simulink model "SimScapeMATE_InductionMachine"  (R2024b)
settings: Solver=FixedStepDiscrete  StartTime=0.0  StopTime=0.5  FixedStep=Ts  RelTol=1e-4
PostLoadFcn:
  | Ts=25e-6;
InitFcn:
  | Ts=25e-6;
undefined symbols (not defined in the file): DiscIntNeverNeededParam
libraries: fl_lib x26, ee_lib x16, nesl_utility x13, spspowerguiLib x1
Description:
  | Copyright 2008-2010 The MathWorks, Inc.
settings Model: ARTEMISmethode_block_infos=$$__separator__$$  Creator=MathWorks  LastModifiedBy=CD8435
settings SolverCC: ZeroCrossAlgorithm=Adaptive  AlgebraicLoopSolver=TrustRegion
settings DataIOCC: SaveFormat=Array  SignalLoggingSaveFormat=ModelDataLogs  ReturnWorkspaceOutputs=off  SignalLoggingName=sigsOut  OutputTimes=[0:1/20:10]
settings OptimizationCC: BlockReduction=off  BooleanDataType=off  ExpressionDepthLimit=2147483647  InitFltsAndDblsToZero=on  EfficientMapNaN2IntZero=off  LifeSpan=inf
settings DebuggingCC: UnderspecifiedInitializationDetection=Classic  MergeDetectMultiDrivingBlocksExec=none  CheckExecutionContextPreStartOutputMsg=on  SignalResolutionControl=TryResolveAllWithWarning  IgnoredZcDiagnostic=none  MultiTaskDSMMsg=warning  MultiTaskCondExecSysMsg=none  SigSpecEnsureSampleTimeMsg=none  FcnCallInpInsideContextMsg=warning  AllowSymbolicDim=off  StateNameClashWarn=warning  SFUnexpectedBacktrackingDiag=warning  SFNoUnconditionalDefaultTransitionDiag=warning  SFExecutionAtInitializationDiag=none  ArithmeticOperatorsInVariantConditions=warning
settings HardwareCC: ProdBitPerPointer=32  ProdBitPerSizeT=32  ProdBitPerPtrDiffT=32  ProdLargestAtomicFloat=None  ProdIntDivRoundTo=Undefined  ProdEndianess=Unspecified  ProdWordSize=32  ProdHWDeviceType=Specified  TargetUnknown=on
settings ModelReferenceCC: EnableRefExpFcnMdlSchedulingChecks=on  PropagateSignalLabelsOutOfModel=off
settings SFSimCC: SimUseLocalCustomCode=off  CustomCodeUndefinedFunction=UseInterfaceOnly
settings RTWCC: RTWUseLocalCustomCode=off  GPUComputeCapability=3.5
settings CodeAppCC: StateflowObjectComments=on
settings GRTTargetCC: TargetFcnLib=ansi_tfl_tmw.mat  TargetLangStandard=C89/C90 (ANSI)  CombineOutputUpdateFcns=off  GRTInterface=on
settings ConfigComp: CovMetricSettings=dw  CovSaveCumulativeToWorkspaceVar=on  CovSaveSingleToWorkspaceVar=on  CovExternalEMLEnable=off
settings SimscapeCC: SimscapeNormalizeSystem=off

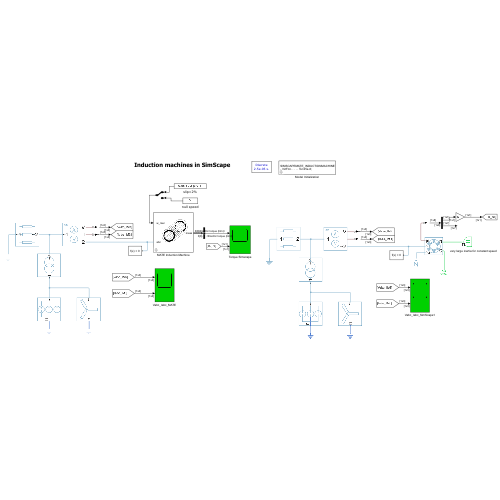
[thumbnail: Simulink's stored preview of the top-level diagram]
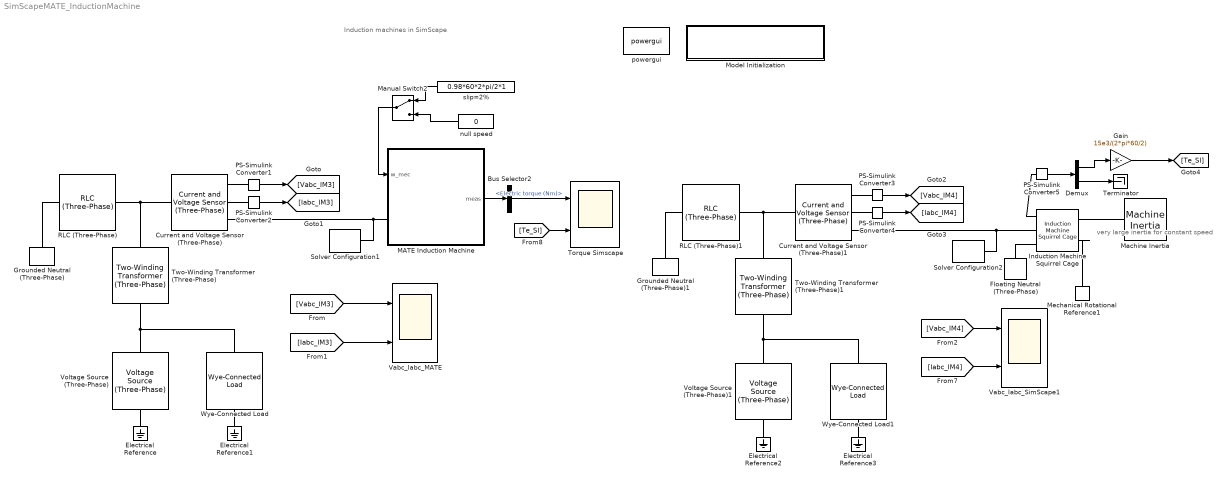
== system SimScapeMATE_InductionMachine ==
  note: very large inertia for constant speed
  note: Induction machines in SimScape
  Bus Selector2 : BusSelector  OutputSignals=Electric torque (Nm)
  Current and Voltage Sensor (Three-Phase) : ee_lib/Sensors & Transducers/Current and Voltage Sensor (Three-Phase)  vMeasurementType=ee.enum.vmeasurement.lg  outputUnit=ee.enum.unit.si  SRated=100e6 A*V  VRated=24e3 V  I_specify=off  I_priority=None  I=[0, 0, 0] A  I_nominal_specify=off  I_nominal_value=1  I_nominal_unit=A  V_specify=off  V_priority=None  V=[0, 0, 0] V  V_nominal_specify=off  V_nominal_value=1  V_nominal_unit=V
      settings: InternalSimscapePortConfiguration="{\"Bottom\":[],\"Left\":[{\"id\":\"N1\",\"label\":\"~1\",\"type\":\"foundation.electrical.three_phase\"}],\"Right\":[{\"id\":\"V_output\",\"label\":\"V\",\"type\":\"output\"},{\"id\":\"I_output\",\"label\":\"I\",\"type\":\"output\"},{\"id\":\"N2\",\"label\":\"~2\",\"type\":\"foundation.electrical.three_phase\"}],\"Top\":[]}"
  Current and Voltage Sensor (Three-Phase)1 : ee_lib/Sensors & Transducers/Current and Voltage Sensor (Three-Phase)  vMeasurementType=ee.enum.vmeasurement.lg  outputUnit=ee.enum.unit.si  SRated=100e6 A*V  VRated=24e3 V  I_specify=off  I_priority=None  I=[0, 0, 0] A  I_nominal_specify=off  I_nominal_value=1  I_nominal_unit=A  V_specify=off  V_priority=None  V=[0, 0, 0] V  V_nominal_specify=off  V_nominal_value=1  V_nominal_unit=V
      settings: InternalSimscapePortConfiguration="{\"Bottom\":[],\"Left\":[{\"id\":\"N1\",\"label\":\"~1\",\"type\":\"foundation.electrical.three_phase\"}],\"Right\":[{\"id\":\"V_output\",\"label\":\"V\",\"type\":\"output\"},{\"id\":\"I_output\",\"label\":\"I\",\"type\":\"output\"},{\"id\":\"N2\",\"label\":\"~2\",\"type\":\"foundation.electrical.three_phase\"}],\"Top\":[]}"
  Demux : Demux  Outputs=[1 -1]
  Electrical Reference{,1..3} (4 alike) : fl_lib/Electrical/Electrical Elements/Electrical Reference
  Floating Neutral (Three-Phase) : ee_lib/Connectors & References/Floating Neutral (Three-Phase)  G_parasitic=1e-12 1/Ohm
      settings: InternalSimscapePortConfiguration="{\"Bottom\":[],\"Left\":[{\"id\":\"N\",\"label\":\"~\",\"type\":\"foundation.electrical.three_phase\"}],\"Right\":[],\"Top\":[]}"
  Gain : Gain  Gain=15e3/(2*pi*60/2)
  Grounded Neutral (Three-Phase) : ee_lib/Connectors & References/Grounded Neutral (Three-Phase)
  Grounded Neutral (Three-Phase)1 : ee_lib/Connectors & References/Grounded Neutral (Three-Phase)
  Induction Machine Squirrel Cage : ee_lib/Electromechanical/Asynchronous/Induction Machine Squirrel Cage  port_option=ee.enum.threePhasePort.composite  SRated=15e3 A*V  VRated=220 V  FRated=60 Hz  nPolePairs=2  param_unit=ee.enum.unit.si  squirrel_cage=ee.enum.squirrelcage.Single  zero_sequence=ee.enum.park.zerosequence.exclude  initialization_option=ee.enum.asm.initialization.fluxvariables  Rs=0.5968 Ohm  Xls=0.0003495*(2*pi*60) Ohm  pu_Rs=0.0258  pu_Lls=0.0413  Rrd=0.6258 Ohm  Xlrd=0.005473*(2*pi*60) Ohm  pu_Rrd=0.0145  pu_Llrd=0.0424  Rrd1=0.28 Ohm  Xlrd1=0.82 Ohm  Rrd2=0.28 Ohm  Xlrd2=0.82 Ohm  pu_Rrd1=0.0290  pu_Llrd1=0.0848  pu_Rrd2=0.0290  pu_Llrd2=0.0848  Xm=0.0354*(2*pi*60) Ohm  pu_Lm=1.7562  X0=0.4 Ohm  pu_L0=0.0413  saturation_option=ee.enum.saturation.exclude  saturation_i=[0, 4, 9, 18, 25, 34, 50, 68, 95, 120] A  saturation_v=[0, 88, 154, 198, 220, 242, 264, 286, 308, 327] V  pu_saturation_i=[0, .176, .396, .792, 1.1, 1.496, 2.2, 2.992, 4.18, 5.28]  pu_saturation_v=[0, .4, .7, .9, 1, 1.1, 1.2, 1.3, 1.4, 1.4864]  connection_option=ee.enum.Connection.delta  angular_position_specify=off  angular_position_priority=None  angular_position=0 deg  angular_position_nominal_specify=off  angular_position_nominal_value=1  angular_position_nominal_unit=deg  pu_psids_specify=off  pu_psids_priority=None  pu_psids=0  pu_psids_nominal_specify=off  pu_psids_nominal_value=1  pu_psids_nominal_unit=1  pu_psiqs_specify=off  pu_psiqs_priority=None  pu_psiqs=0  pu_psiqs_nominal_specify=off  pu_psiqs_nominal_value=1  pu_psiqs_nominal_unit=1  pu_psi0s_specify=off  pu_psi0s_priority=None  pu_psi0s=0  pu_psi0s_nominal_specify=off  pu_psi0s_nominal_value=1  pu_psi0s_nominal_unit=1  pu_psidr_specify=off  pu_psidr_priority=None  pu_psidr=0  pu_psidr_nominal_specify=off  pu_psidr_nominal_value=1  pu_psidr_nominal_unit=1  pu_psiqr_specify=off  pu_psiqr_priority=None  pu_psiqr=0  pu_psiqr_nominal_specify=off  pu_psiqr_nominal_value=1  pu_psiqr_nominal_unit=1  pu_psidr1_specify=off  pu_psidr1_priority=None  pu_psidr1=0  pu_psidr1_nominal_specify=off  pu_psidr1_nominal_value=1  pu_psidr1_nominal_unit=1  pu_psiqr1_specify=off  pu_psiqr1_priority=None  pu_psiqr1=0  pu_psiqr1_nominal_specify=off  pu_psiqr1_nominal_value=1  pu_psiqr1_nominal_unit=1  pu_psidr2_specify=off  pu_psidr2_priority=None  pu_psidr2=0  pu_psidr2_nominal_specify=off  pu_psidr2_nominal_value=1  pu_psidr2_nominal_unit=1  pu_psiqr2_specify=off  pu_psiqr2_priority=None  pu_psiqr2=0  pu_psiqr2_nominal_specify=off  pu_psiqr2_nominal_value=1  pu_psiqr2_nominal_unit=1  psids_specify=off  psids_priority=None  psids=0 Wb  psids_nominal_specify=off  psids_nominal_value=1  psids_nominal_unit=Wb  psiqs_specify=off  psiqs_priority=None  psiqs=0 Wb  psiqs_nominal_specify=off  psiqs_nominal_value=1  psiqs_nominal_unit=Wb  psi0s_specify=off  psi0s_priority=None  psi0s=0 Wb  psi0s_nominal_specify=off  psi0s_nominal_value=1  psi0s_nominal_unit=Wb  psidr_specify=off  psidr_priority=None  psidr=0 Wb  psidr_nominal_specify=off  psidr_nominal_value=1  psidr_nominal_unit=Wb  psiqr_specify=off  psiqr_priority=None  psiqr=0 Wb  psiqr_nominal_specify=off  psiqr_nominal_value=1  psiqr_nominal_unit=Wb  psidr1_specify=off  psidr1_priority=None  psidr1=0 Wb  psidr1_nominal_specify=off  psidr1_nominal_value=1  psidr1_nominal_unit=Wb  psiqr1_specify=off  psiqr1_priority=None  psiqr1=0 Wb  psiqr1_nominal_specify=off  psiqr1_nominal_value=1  psiqr1_nominal_unit=Wb  psidr2_specify=off  psidr2_priority=None  psidr2=0 Wb  psidr2_nominal_specify=off  psidr2_nominal_value=1  psidr2_nominal_unit=Wb  psiqr2_specify=off  psiqr2_priority=None  psiqr2=0 Wb  psiqr2_nominal_specify=off  psiqr2_nominal_value=1  psiqr2_nominal_unit=Wb  slip_specify=off  slip_priority=None  slip=0  slip_nominal_specify=off  slip_nominal_value=1  slip_nominal_unit=1  real_power_generated_specify=off  real_power_generated_priority=None  real_power_generated=0 W  real_power_generated_nominal_specify=off  real_power_generated_nominal_value=1  real_power_generated_nominal_unit=W  mechanical_power_consumed_specify=off  mechanical_power_consumed_priority=None  mechanical_power_consumed=0 W  mechanical_power_consumed_nominal_specify=off  mechanical_power_consumed_nominal_value=1  mechanical_power_consumed_nominal_unit=W  Tmeas=298.15 K  alpha=3.93e-3 1/K  alpha_cage=4.4e-3 1/K  stator_thermal_mass=100 J/K  rotor_thermal_mass=200 J/K  temperatureA_specify=off  temperatureA_priority=High  temperatureA=25 degC  temperatureA_nominal_specify=off  temperatureA_nominal_value=1  temperatureA_nominal_unit=degC  temperatureB_specify=off  temperatureB_priority=High  temperatureB=25 degC  temperatureB_nominal_specify=off  temperatureB_nominal_value=1  temperatureB_nominal_unit=degC  temperatureC_specify=off  temperatureC_priority=High  temperatureC=25 degC  temperatureC_nominal_specify=off  temperatureC_nominal_value=1  temperatureC_nominal_unit=degC  temperatureR_specify=off  temperatureR_priority=High  temperatureR=25 degC  temperatureR_nominal_specify=off  temperatureR_nominal_value=1  temperatureR_nominal_unit=degC
      settings: InternalSimscapePortConfiguration="{\"Bottom\":[],\"Left\":[{\"id\":\"R\",\"label\":\"R\",\"type\":\"foundation.mechanical.rotational.rotational\"},{\"id\":\"C\",\"label\":\"C\",\"type\":\"foundation.mechanical.rotational.rotational\"}],\"Right\":[{\"id\":\"pu_output\",\"label\":\"pu\",\"type\":\"output\"},{\"id\":\"N1\",\"label\":\"~1\",\"type\":\"foundation.electrical.three_phase\"},{\"id\":\"N2\",\"label\":\"~2\",\"type\":\"foundation.electrical.three_phase\"}],\"Top\":[]}"
  MATE Induction Machine : Subsystem  mask(MATE Induction Machine){Rs=0.5968, Lls=0.0003495, Rr=0.6258, Llr=0.005473, Lm=0.0354, pp=2, Ts=Ts, disc=Backward Euler, park=Rotor, Parameter11=|}
      mask Parameter11=|
      | Induction machine equations in rotor or stationary reference frame:
      |
      |   v = [R]*i + dphi/dt + [W]*phi
      | phi = [L]*i
      |
      | where:
      | [R] = diagonal matrix (4,4) of winding resistances in d q axis
      | [L] = matrix (4,4) of winding self and mutual inductances in d q axis
      | [W] = matrix (4,4) depending on rotor speed wr and reference frame
      |
      |   v = voltage vector      = [vds   vqs   vdr   vqr  ]'
      | phi = flux linkage vector = [phids phiqs phidr phiqr]' (state variables)
      |   i = current vector      = [ids   iqs   idr   iqr  ]'
      |
      | In the discretized model and to provide a constant admittance to the SimScape solver, the speed term [W]*phi is incorporated with a one step delay, so to transform this component into an input to the state equations. This is a very common approach, used in major software like EMTP.
      |
      | The model uses an orthogonal Park transform. Internally, fluxes are scalled differently than the claissic 'Krause' Park transform (with 2/3 factors). Notably, the torque equation has no 3/2 scaling factor, due the power invariability of the orthogonal Park transform.
      |
      | Rotor-based and Fixed reference produces similar accuracy, depending on the operating point. For real-time applications however, the fixed reference frame internal parameters such as the discrete ABCD matrices are constant and do not need to be recomputed at each time step and is therefore faster in simulation.
      mask prompts: Rs "Stator resistance [Ohms]"; Lls "Stator leakeage inductance [H]"; Rr "Rotor resistance (seen from stator) [Ohms]"; Llr "Rotor leakeage inductance (seen from stator) [H]"; Lm "Mutual inductance [H]"; pp "Number of pairs of poles"; Ts "Sample Time (s)"; disc "Discretization"; park "D-Q reference frame"
      mask help:
      | The MATE induction machine implements a three-phase asynchronous machine (squirrel cage) modeled with a fixed or rotot-based dq reference frame. Stator and rotor windings are connected in wye to an internal neutral point.
      |
      | In SimScape, this model provides a constant admittance that can be pre-factorized in the global Jacobian matrix of the SimScape solver. This can lead to speed improvements for real-time applications.
      |
      | Inputs: w_mec: the mechanical frequency of the rotor in rad/s.
      mask init:
      | dis=get_param(gcb,'disc');
      | if isequal(dis,'Backward Euler')
      |     be='on';
      |     ben=1;
      | else
      |     be='off';
      |     ben=0;
      | end
      | 
      | parkk=get_param(gcb,'park');
      | 
      | if isequal(parkk,'Stationary')
      |     park_num=1;
      | else
      |     park_num=0;
      | end
      | 
      | 
      | Lr=Lm+Llr;
      | Ls=Lm+Lls;
      | 
      | invLmat=1/(Lr*Ls-Lm*Lm)*[Lr 0 -Lm 0; 0 Lr 0 -Lm; -Lm 0  Ls  0;  0  -Lm  0  Ls];
      | moinsRmat=-[Rs 0 0 0; 0 Rs 0 0; 0 0  Rr  0;  0  0  0  Rr];
      | 
      | 
      | 
      | T=[1 0;0 1]*sqrt(2/3)*[1 -0.5 -0.5;0 sqrt(3)/2 -sqrt(3)/2];
      | 
      | T=cat(1,T,[0 0 0; 0 0 0]);
      | 
      | if isequal(be,'off')
      |     Bd=Ts/2*inv(eye(4)-Ts/2*moinsRmat*invLmat)*T; %trapeze
      | else
      |     Bd=Ts*inv(eye(4)-Ts*moinsRmat*invLmat)*T;   % euler
      | end
      | 
      | Cd=T'*invLmat;
      | 
      | 
      | Y=Cd*Bd;
      | 
      | % setting external resistances 
      | ResistanceM=zeros(3,3);
      | 
      | Ytot=Y;
      | Yav=(-1/Ytot(1,2)-1/Ytot(1,3)-1/Ytot(2,3))/3;
      | 
      | 
      | ResistanceM(1,2)=Yav;
      | ResistanceM(1,3)=Yav;
      | ResistanceM(2,3)=Yav;
      | 
      | ResistanceM(1,1)=1e12;
      | ResistanceM(2,2)=1e12;
      | ResistanceM(3,3)=1e12;
      mask TypeOptions disc: Backward Euler | Trapezoidal
      mask TypeOptions park: Stationary | Rotor
      mask DialogControl ParameterTabVar0 Prompt: Parameters
      mask DialogControl ParameterTabVar01 Prompt: Advanced parameters
      mask DialogControl Container7 Prompt: More Info
  Machine Inertia : ee_lib/Electromechanical/Mechanical/Machine Inertia  SRated=164000 V*A  FRated=60 Hz  nPolePairs=2  inertia_option=1  J=1e8 kg*m^2  H=0.2734 s*W/V/A  damper_option=2  D=39.0509 N*m/(rad/s)  pu_D=0.0106  initialization_option=1  fMechanical0=0.98*60/2 Hz  fElectrical0=0 Hz
      settings: InternalSimscapePortConfiguration="{\"Bottom\":[],\"Left\":[{\"id\":\"R\",\"label\":\"R\",\"type\":\"foundation.mechanical.rotational.rotational\"}],\"Right\":[],\"Top\":[]}"
  Manual Switch2 : ManualSwitch
  Mechanical Rotational Reference1 : fl_lib/Mechanical/Rotational Elements/Mechanical Rotational Reference
  Model Initialization : Subsystem  mask(Model Functions){InitFcnX=Ts=25e-6;, prel=off, posl=on, inif=on, strf=off}
      mask prompts: InitFcnX "Initialisation"; prel "Preload Function"; posl "PostLoad Function"; inif "InitFcn"; strf "StartFcn"
      mask init:
      | currentBlock = gcb;
      | root = bdroot(currentBlock);
      | 
      | if ~strcmp(get_param(root,'BlockDiagramType'),'library')
      |     if prel==1
      |         set_param(root, 'PreLoadFcn', InitFcnX);
      |     else
      |         set_param(root, 'PreLoadFcn', '');
      |     end
      |     if inif==1
      |         set_param(root, 'InitFcn', InitFcnX);
      |     else
      |         set_param(root, 'InitFcn', '');
      |     end
      |     if strf==1
      |         set_param(root, 'StartFcn', InitFcnX);
      |     else
      |         set_param(root, 'StartFcn', '');
      |     end
      |     if posl==1
      |         set_param(root, 'PostLoadFcn', InitFcnX);
      |     else
      |         set_param(root, 'PostLoadFcn', '');
      |     end
      | end
      | 
      | pos = get_param(currentBlock, 'Position');
      | width = pos(3) - pos(1); height = pos(4) - pos(2);
      | txt = [ upper(root) '\n' '- InitFcn. . . . . '  get_param(root, 'InitFcn') ];
      settings: CopyFcn=set_param(gcb,'LinkStatus','inactive')
      mask Display: text(5, height*0.5, txt, 'horizontalAlignment', 'left', 'verticalAlignment', 'middle') ;
  PS-Simulink Converter{1..5} (5 alike) : nesl_utility/PS-Simulink Converter  PhysicalDomain=network_engine_domain  SubClassName=ps_output  LeftPortType=input  RightPortType=output  PseudoPeriodic=off  Frequencies=[]  VectorFormat=inherit  Unit=inherit  AffineConversion=off
  RLC (Three-Phase) : ee_lib/Passive/RLC Assemblies/RLC (Three-Phase)  port_option=ee.enum.threePhasePort.composite  component_structure=ee.enum.rlc.structure.R  R=1e7 Ohm  L=1e-3 H  C=1e-6 F  R_parasitic=0 Ohm  G_parasitic=0 1/Ohm  IL_specify=off  IL_priority=High  IL=[0, 0, 0] A  IL_nominal_specify=off  IL_nominal_value=1  IL_nominal_unit=A  VC_specify=off  VC_priority=High  VC=[0, 0, 0] V  VC_nominal_specify=off  VC_nominal_value=1  VC_nominal_unit=V
      settings: InternalSimscapePortConfiguration="{\"Bottom\":[],\"Left\":[{\"id\":\"N1\",\"label\":\"~1\",\"type\":\"foundation.electrical.three_phase\"}],\"Right\":[{\"id\":\"N2\",\"label\":\"~2\",\"type\":\"foundation.electrical.three_phase\"}],\"Top\":[]}"
  RLC (Three-Phase)1 : ee_lib/Passive/RLC Assemblies/RLC (Three-Phase)  port_option=ee.enum.threePhasePort.composite  component_structure=ee.enum.rlc.structure.R  R=1e7 Ohm  L=1e-3 H  C=1e-6 F  R_parasitic=0 Ohm  G_parasitic=0 1/Ohm  IL_specify=off  IL_priority=High  IL=[0, 0, 0] A  IL_nominal_specify=off  IL_nominal_value=1  IL_nominal_unit=A  VC_specify=off  VC_priority=High  VC=[0, 0, 0] V  VC_nominal_specify=off  VC_nominal_value=1  VC_nominal_unit=V
      settings: InternalSimscapePortConfiguration="{\"Bottom\":[],\"Left\":[{\"id\":\"N1\",\"label\":\"~1\",\"type\":\"foundation.electrical.three_phase\"}],\"Right\":[{\"id\":\"N2\",\"label\":\"~2\",\"type\":\"foundation.electrical.three_phase\"}],\"Top\":[]}"
  Solver Configuration1 : nesl_utility/Solver Configuration  PhysicalDomain=network_engine_domain  SubClassName=solver  LeftPortType=input  RightPortType=generic  Tones=[]  Harmonics=[]  SimulateNoise=off  Profile=off  UseLocalSampling=off  EnableSwitchedLinearOptims=on  FrequencyDomain=off  UseCCode=off  RelTol=0.001  AbsTol=1e-06  MinStep=1e-09  ToWorkspace=off  RevertToSquareIcSolve=off  NumHomotopyIterations=100  PhasorMode=off  PhasorModeNumHarmonics=1  ConsistencySolver=NEWTON_FTOL  IndexReductionMethod=DerivativeReplacement  DoDC=off  ResidualTolerance=0.001  ConsistencyTolSource=GLOBAL  ConsistencyAbsTol=0.001  ConsistencyRelTol=0.001  ConsistencyTolFactor=0.001  UseLocalSolver=on  LocalSolverChoice=NE_BACKWARD_EULER_ADVANCER  ResolveIndetEquations=off  FunctionEvalNumThread=1  LocalSolverSampleTime=Ts  DoFixedCost=on  MaxNonlinIter=1  MaxModeIter=2  ComputeImpulses=off  ImpulseIterations=2  LinearAlgebra=Sparse  LinearAlgebraNumThread=0  EquationFormulation=NE_TIME_EF  DelaysMemoryBudget=1024  AutomaticFiltering=off  FilteringTimeConstant=0.001  PartitionStorageMethod=AS_NEEDED  PartitionMemoryBudget=1024  PartitionMethod=ROBUST  MultibodyUseLocalSolver=off  MultibodyLocalSolverChoice=ODE1  MultibodyLocalSolverSampleTime=0.001
  Solver Configuration2 : nesl_utility/Solver Configuration  PhysicalDomain=network_engine_domain  SubClassName=solver  LeftPortType=input  RightPortType=generic  Tones=[]  Harmonics=[]  SimulateNoise=off  Profile=off  UseLocalSampling=off  EnableSwitchedLinearOptims=on  FrequencyDomain=off  UseCCode=off  RelTol=0.001  AbsTol=1e-06  MinStep=1e-09  ToWorkspace=off  RevertToSquareIcSolve=off  NumHomotopyIterations=100  PhasorMode=off  PhasorModeNumHarmonics=1  ConsistencySolver=NEWTON_FTOL  IndexReductionMethod=DerivativeReplacement  DoDC=off  ResidualTolerance=0.001  ConsistencyTolSource=GLOBAL  ConsistencyAbsTol=0.001  ConsistencyRelTol=0.001  ConsistencyTolFactor=0.001  UseLocalSolver=on  LocalSolverChoice=NE_BACKWARD_EULER_ADVANCER  ResolveIndetEquations=off  FunctionEvalNumThread=1  LocalSolverSampleTime=Ts  DoFixedCost=on  MaxNonlinIter=1  MaxModeIter=2  ComputeImpulses=off  ImpulseIterations=2  LinearAlgebra=Sparse  LinearAlgebraNumThread=0  EquationFormulation=NE_TIME_EF  DelaysMemoryBudget=1024  AutomaticFiltering=off  FilteringTimeConstant=0.001  PartitionStorageMethod=AS_NEEDED  PartitionMemoryBudget=1024  PartitionMethod=ROBUST  MultibodyUseLocalSolver=off  MultibodyLocalSolverChoice=ODE1  MultibodyLocalSolverSampleTime=0.001
  Terminator : Terminator
  Torque Simscape : Scope  NumInputPorts=2
  Two-Winding Transformer (Three-Phase) : ee_lib/Passive/Transformers/Two-Winding Transformer (Three-Phase)  SRated=6e6 A*V  FRated=60 Hz  Winding1Connection=ee.enum.windingconnection.Yg  VRated1=25e3 V  Winding2Connection=ee.enum.windingconnection.delta1  VRated2=2400 V  CoreType=ee.enum.coretype.threelimb  pu_Rw1=0.0015  pu_Rw2=0.0015  leakage_reactance_option=ee.enum.transformer_leakage.include  pu_Xl1=0.03  pu_Xl2=0.03  magnetizing_resistance_option=ee.enum.transformer_magnetizingResistance.include  pu_Rm=200  magnetizing_reactance_option=ee.enum.transformer_magnetizingReactance.include  saturation_option=ee.enum.transformer_saturation.exclude  pu_Xm=200  current_data=[0, .002, 1, 2]  magnetic_flux_data=[0, 1.2, 1.5, 1.51]  pu_X0=0.5  i1_specify=on  i1_priority=High  i1=[0, 0, 0] A  i1_nominal_specify=off  i1_nominal_value=1  i1_nominal_unit=A  i2_specify=on  i2_priority=High  i2=[0, 0, 0] A  i2_nominal_specify=off  i2_nominal_value=1  i2_nominal_unit=A  phi_specify=off  phi_priority=None  phi=[0, 0, 0]  phi_nominal_specify=off  phi_nominal_value=1  phi_nominal_unit=1  power_dissipated_specify=off  power_dissipated_priority=None  power_dissipated=0 W  power_dissipated_nominal_specify=off  power_dissipated_nominal_value=1  power_dissipated_nominal_unit=W
      settings: InternalSimscapePortConfiguration="{\"Bottom\":[],\"Left\":[{\"id\":\"N1\",\"label\":\"~1\",\"type\":\"foundation.electrical.three_phase\"}],\"Right\":[{\"id\":\"N2\",\"label\":\"~2\",\"type\":\"foundation.electrical.three_phase\"}],\"Top\":[]}"
  Two-Winding Transformer (Three-Phase)1 : ee_lib/Passive/Transformers/Two-Winding Transformer (Three-Phase)  SRated=6e6 A*V  FRated=60 Hz  Winding1Connection=ee.enum.windingconnection.Yg  VRated1=25e3 V  Winding2Connection=ee.enum.windingconnection.delta1  VRated2=2400 V  CoreType=ee.enum.coretype.threelimb  pu_Rw1=0.0015  pu_Rw2=0.0015  leakage_reactance_option=ee.enum.transformer_leakage.include  pu_Xl1=0.03  pu_Xl2=0.03  magnetizing_resistance_option=ee.enum.transformer_magnetizingResistance.include  pu_Rm=200  magnetizing_reactance_option=ee.enum.transformer_magnetizingReactance.include  saturation_option=ee.enum.transformer_saturation.exclude  pu_Xm=200  current_data=[0, .002, 1, 2]  magnetic_flux_data=[0, 1.2, 1.5, 1.51]  pu_X0=0.5  i1_specify=on  i1_priority=High  i1=[0, 0, 0] A  i1_nominal_specify=off  i1_nominal_value=1  i1_nominal_unit=A  i2_specify=on  i2_priority=High  i2=[0, 0, 0] A  i2_nominal_specify=off  i2_nominal_value=1  i2_nominal_unit=A  phi_specify=off  phi_priority=None  phi=[0, 0, 0]  phi_nominal_specify=off  phi_nominal_value=1  phi_nominal_unit=1  power_dissipated_specify=off  power_dissipated_priority=None  power_dissipated=0 W  power_dissipated_nominal_specify=off  power_dissipated_nominal_value=1  power_dissipated_nominal_unit=W
      settings: InternalSimscapePortConfiguration="{\"Bottom\":[],\"Left\":[{\"id\":\"N1\",\"label\":\"~1\",\"type\":\"foundation.electrical.three_phase\"}],\"Right\":[{\"id\":\"N2\",\"label\":\"~2\",\"type\":\"foundation.electrical.three_phase\"}],\"Top\":[]}"
  Vabc_Iabc_MATE : Scope  NumInputPorts=2
  Vabc_Iabc_SimScape1 : Scope  NumInputPorts=2
  Voltage Source (Three-Phase) : ee_lib/Sources/Voltage Source (Three-Phase)  vline_rms=(25000)*1.00135 V  shift=0 deg  freq=60 Hz  impedance_option=4  SShortCircuit=1000e6 A*V  XR=10  R=0.8 Ohm  L=1e-3 H  harmonic_option=0  harmonic_orders=[5, 7, 11, 13]  harmonic_ratios=[.1, .1, .1, .1]  G_parasitic=0 1/Ohm  I_specify=off  I_priority=None  I=[0, 0, 0] A  I_nominal_specify=off  I_nominal_value=1  I_nominal_unit=A
  Voltage Source (Three-Phase)1 : ee_lib/Sources/Voltage Source (Three-Phase)  vline_rms=(25000)*1.00135 V  shift=0 deg  freq=60 Hz  impedance_option=4  SShortCircuit=1000e6 A*V  XR=10  R=0.8 Ohm  L=1e-3 H  harmonic_option=0  harmonic_orders=[5, 7, 11, 13]  harmonic_ratios=[.1, .1, .1, .1]  G_parasitic=0 1/Ohm  I_specify=off  I_priority=None  I=[0, 0, 0] A  I_nominal_specify=off  I_nominal_value=1  I_nominal_unit=A
  Wye-Connected Load : ee_lib/Passive/RLC Assemblies/Wye-Connected Load  port_option=ee.enum.threePhasePort.composite  parameterization=ee.enum.rlc.parameterization.ratedpower  component_structure=ee.enum.rlc.structure.R  component_structure_PQ=ee.enum.rlc.structure.R  R=1 Ohm  L=1e-3 H  C=1e-6 F  VRated=25e3 V  FRated=60 Hz  P=5e6 W  Qpos=1e2 A*V  Qneg=-1e2 A*V  R_parasitic=1e-6 Ohm  G_parasitic=1e-6 1/Ohm  R_parasitic_PQ=1e-6 Ohm  G_parasitic_PQ=1e-6 1/Ohm  Vmag0=24e3 V  Vang0=0 deg  Freq0=60 Hz  IL_specify=off  IL_priority=High  IL=[0, 0, 0] A  IL_nominal_specify=off  IL_nominal_value=1  IL_nominal_unit=A  VC_specify=off  VC_priority=High  VC=[0, 0, 0] V  VC_nominal_specify=off  VC_nominal_value=1  VC_nominal_unit=V
  Wye-Connected Load1 : ee_lib/Passive/RLC Assemblies/Wye-Connected Load  port_option=ee.enum.threePhasePort.composite  parameterization=ee.enum.rlc.parameterization.ratedpower  component_structure=ee.enum.rlc.structure.R  component_structure_PQ=ee.enum.rlc.structure.R  R=1 Ohm  L=1e-3 H  C=1e-6 F  VRated=25e3 V  FRated=60 Hz  P=5e6 W  Qpos=1e2 A*V  Qneg=-1e2 A*V  R_parasitic=1e-6 Ohm  G_parasitic=1e-6 1/Ohm  R_parasitic_PQ=1e-6 Ohm  G_parasitic_PQ=1e-6 1/Ohm  Vmag0=24e3 V  Vang0=0 deg  Freq0=60 Hz  IL_specify=off  IL_priority=High  IL=[0, 0, 0] A  IL_nominal_specify=off  IL_nominal_value=1  IL_nominal_unit=A  VC_specify=off  VC_priority=High  VC=[0, 0, 0] V  VC_nominal_specify=off  VC_nominal_value=1  VC_nominal_unit=V
  null speed : Constant  Value=0
  powergui : spspowerguiLib/powergui  Priority=1  SimulationMode=Discrete  SampleTime=Ts  frequency=60  Iterations=50  frequencyindice=60  Pbase=100e6  ErrMax=1e-4  UnitsV=kV  UnitsW=MW  buscounter=0  FunctionMessages=off  echomessages=off  EnableUseOfTLC=off  CurrentSourceSwitches=off  DisableSnubberDevices=off  DisableRonSwitches=off  DisableVfSwitches=off  DisplayEquations=off  AutomaticDiscreteSolvers=off  SolverType=Tustin  Interpol=off  ExternalGateDelay=off  methode=off  Ts=10  x0status=zero  SPID=off  SwTol=0  HookPort=off  NonlinearTolerance=1e-4  nMaxIteration=100  ContinueOnMaxIteration=off  RestoreLinks=warning  ResistiveCurrentMeasurement=off  Frange=[0:2:500]  Ylog=off  Xlog=on  ShowGrid=off  save=off  variable=ZData  structure=0  ZoomFFT=off  StartTime=0.0  cycles=1  DisplayStyle=1  fundamental=60  FreqAxis=off  MaxFrequency=1000  frequencyindicesteady=1  RmsSteady=1  display=off
  slip=2% : Constant  Value=0.98*60*2*pi/2*1
  wires:
  Bus Selector2/1 -> Torque Simscape/1  "<Electric torque (Nm)>"
  MATE Induction Machine/1(meas) -> Bus Selector2/1
  slip=2%/1 -> Manual Switch2/1
  null speed/1 -> Manual Switch2/2
  Manual Switch2/1 -> MATE Induction Machine/1("   w_mec")
  PS-Simulink Converter1/1 -> [Vabc_IM3]
  PS-Simulink Converter2/1 -> [Iabc_IM3]
  [Iabc_IM3] -> Vabc_Iabc_MATE/2
  [Vabc_IM3] -> Vabc_Iabc_MATE/1
  [Vabc_IM4] -> Vabc_Iabc_SimScape1/1
  [Iabc_IM4] -> Vabc_Iabc_SimScape1/2
  PS-Simulink Converter4/1 -> [Iabc_IM4]
  PS-Simulink Converter3/1 -> [Vabc_IM4]
  PS-Simulink Converter5/1 -> Demux/1
  Demux/1 -> Gain/1
  Gain/1 -> [Te_SI]
  [Te_SI] -> Torque Simscape/2
  Demux/2 -> Terminator/1
  connections:
  Electrical Reference/LConn1 -- Voltage Source (Three-Phase)/LConn1
  Voltage Source (Three-Phase)/RConn1 -- Wye-Connected Load/LConn1 -- Two-Winding Transformer (Three-Phase)/LConn1
  Two-Winding Transformer (Three-Phase)/RConn1 -- RLC (Three-Phase)/RConn1 -- Current and Voltage Sensor (Three-Phase)/LConn1
  Current and Voltage Sensor (Three-Phase)/RConn3 -- Solver Configuration1/RConn1 -- MATE Induction Machine/LConn1
  PS-Simulink Converter2/LConn1 -- Current and Voltage Sensor (Three-Phase)/RConn2
  PS-Simulink Converter1/LConn1 -- Current and Voltage Sensor (Three-Phase)/RConn1
  Electrical Reference1/LConn1 -- Wye-Connected Load/RConn1
  Grounded Neutral (Three-Phase)/LConn1 -- RLC (Three-Phase)/LConn1
  Wye-Connected Load1/LConn1 -- Voltage Source (Three-Phase)1/RConn1 -- Two-Winding Transformer (Three-Phase)1/LConn1
  Two-Winding Transformer (Three-Phase)1/RConn1 -- Current and Voltage Sensor (Three-Phase)1/LConn1 -- RLC (Three-Phase)1/RConn1
  Current and Voltage Sensor (Three-Phase)1/RConn3 -- Induction Machine Squirrel Cage/RConn2 -- Solver Configuration2/RConn1
  PS-Simulink Converter3/LConn1 -- Current and Voltage Sensor (Three-Phase)1/RConn1
  PS-Simulink Converter4/LConn1 -- Current and Voltage Sensor (Three-Phase)1/RConn2
  Electrical Reference3/LConn1 -- Wye-Connected Load1/RConn1
  Grounded Neutral (Three-Phase)1/LConn1 -- RLC (Three-Phase)1/LConn1
  Electrical Reference2/LConn1 -- Voltage Source (Three-Phase)1/LConn1
  Floating Neutral (Three-Phase)/LConn1 -- Induction Machine Squirrel Cage/RConn3
  Induction Machine Squirrel Cage/LConn1 -- Machine Inertia/LConn1
  Induction Machine Squirrel Cage/LConn2 -- Mechanical Rotational Reference1/LConn1
  Induction Machine Squirrel Cage/RConn1 -- PS-Simulink Converter5/LConn1

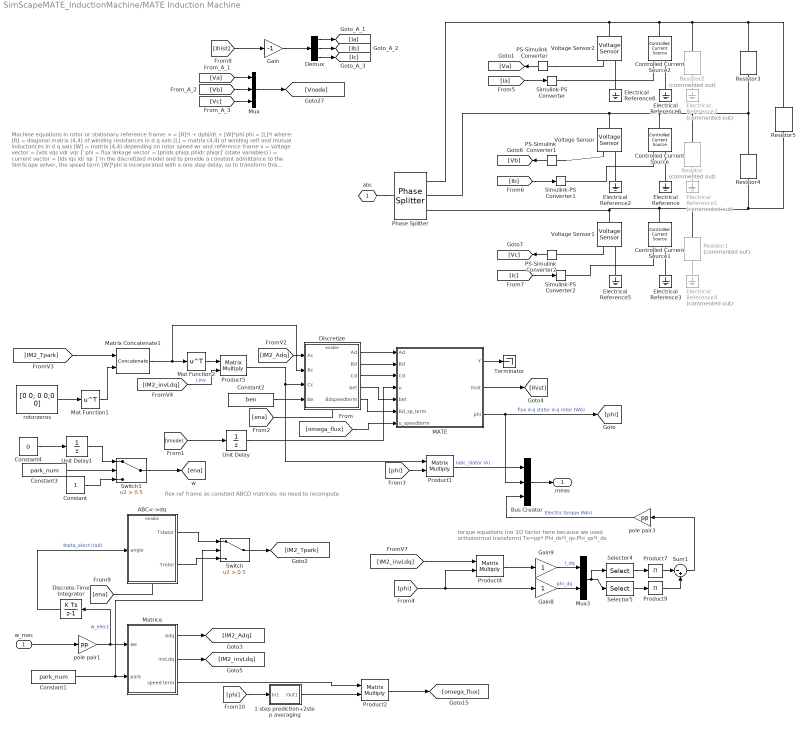
== system SimScapeMATE_InductionMachine/MATE Induction Machine ==
  note: fiex ref frame as constant ABCD matrices: no need to recompute
  note: torque equations
      | (no 3/2 factor here because we used orthonormal transform)
      | Te=pp* Phi_ds*I_qs-Phi_qs*I_ds
  note: Machine equations in rotor or stationary reference frame:
      |
      |   v = [R]*i + dphi/dt + [W]*phi
      | phi = [L]*i
      |
      | where:
      | [R] = diagonal matrix (4,4) of winding resistances in d q axis
      | [L] = matrix (4,4) of winding self and mutual inductances in d q axis
      | [W] = matrix (4,4) depending on rotor speed wr and reference frame
      |
      |   v = voltage vector      = [vds   vqs   vdr   vqr  ]'
      | phi = flux linkage vector = [phids phiqs phidr phiqr]' (state variables)
      |   i = current vector      = [ids   iqs   idr   iqr  ]'
      |
      | In the discretized model and to provide a constant admittance to the SimScape solver, the speed term [W]*phi is incorporated with a one step delay, so to transform this component into an input to the state equations
  "   w_mec" : Inport
  1 step prediction+2step averaging : Subsystem
  ABC<->dq : Subsystem
  Bus Creator : BusCreator  Inputs=3
  Constant : Constant
  Constant1 : Constant  Value=park_num
  Constant2 : Constant  Value=ben
  Constant3 : Constant  Value=park_num
  Constant4 : Constant  Value=0
  Controlled Current Source : fl_lib/Electrical/Electrical Sources/Controlled Current Source
  Controlled Current Source1 : fl_lib/Electrical/Electrical Sources/Controlled Current Source
  Controlled Current Source2 : fl_lib/Electrical/Electrical Sources/Controlled Current Source
  Demux : Demux  Outputs=3
      settings: DisplayOption=none
  Discrete-Time Integrator : DiscreteIntegrator  SampleTime=Ts  ICPrevOutput=DiscIntNeverNeededParam  ICPrevScaledInput=DiscIntNeverNeededParam
  Discretize : Subsystem
  Electrical Reference{,2..3,5..6,8} (6 alike) : fl_lib/Electrical/Electrical Elements/Electrical Reference
  Electrical Reference1 : fl_lib/Electrical/Electrical Elements/Electrical Reference  Commented=on
  Electrical Reference4 : fl_lib/Electrical/Electrical Elements/Electrical Reference  Commented=on
  Electrical Reference7 : fl_lib/Electrical/Electrical Elements/Electrical Reference  Commented=on
  Gain : Gain  Gain=-1
  Gain8 : Gain
  Gain9 : Gain
  MATE : Subsystem
  Mat Function1 : Math  Operator=transpose  SignedPower=on
  Mat Function2 : Math  Operator=transpose  SignedPower=on
  Matrice : Subsystem
  Matrix Concatenate1 : Concatenate  Mode=Multidimensional array
  Mux : Mux  Inputs=3
  Mux3 : Mux  Inputs=2
  PS-Simulink Converter : nesl_utility/PS-Simulink Converter  PhysicalDomain=network_engine_domain  SubClassName=ps_output  LeftPortType=input  RightPortType=output  PseudoPeriodic=off  Frequencies=[]  VectorFormat=inherit  Unit=inherit  AffineConversion=off
  PS-Simulink Converter1 : nesl_utility/PS-Simulink Converter  PhysicalDomain=network_engine_domain  SubClassName=ps_output  LeftPortType=input  RightPortType=output  PseudoPeriodic=off  Frequencies=[]  VectorFormat=inherit  Unit=inherit  AffineConversion=off
  PS-Simulink Converter2 : nesl_utility/PS-Simulink Converter  PhysicalDomain=network_engine_domain  SubClassName=ps_output  LeftPortType=input  RightPortType=output  PseudoPeriodic=off  Frequencies=[]  VectorFormat=inherit  Unit=inherit  AffineConversion=off
  Phase Splitter : ee_lib/Connectors & References/Phase Splitter
  Product{1..2,4..5} (4 alike) : Product  Multiplication=Matrix(*)  SaturateOnIntegerOverflow=on  OutDataTypeStr=Inherit: Same as first input
  Product7 : Product  Inputs=1  InputSameDT=on  SaturateOnIntegerOverflow=on  OutDataTypeStr=Inherit: Same as first input
  Product9 : Product  Inputs=1  InputSameDT=on  SaturateOnIntegerOverflow=on  OutDataTypeStr=Inherit: Same as first input
  Resistor : fl_lib/Electrical/Electrical Elements/Resistor  Commented=on  R=ResistanceM(2,2) Ohm  i_specify=off  i_priority=None  i=0 A  i_nominal_specify=off  i_nominal_value=1  i_nominal_unit=A  v_specify=off  v_priority=None  v=0 V  v_nominal_specify=off  v_nominal_value=1  v_nominal_unit=V
  Resistor1 : fl_lib/Electrical/Electrical Elements/Resistor  Commented=on  R=ResistanceM(3,3) Ohm  i_specify=off  i_priority=None  i=0 A  i_nominal_specify=off  i_nominal_value=1  i_nominal_unit=A  v_specify=off  v_priority=None  v=0 V  v_nominal_specify=off  v_nominal_value=1  v_nominal_unit=V
  Resistor2 : fl_lib/Electrical/Electrical Elements/Resistor  Commented=on  R=ResistanceM(1,1) Ohm  i_specify=off  i_priority=None  i=0 A  i_nominal_specify=off  i_nominal_value=1  i_nominal_unit=A  v_specify=off  v_priority=None  v=0 V  v_nominal_specify=off  v_nominal_value=1  v_nominal_unit=V
  Resistor3 : fl_lib/Electrical/Electrical Elements/Resistor  R=ResistanceM(1,2) Ohm  i_specify=off  i_priority=None  i=0 A  i_nominal_specify=off  i_nominal_value=1  i_nominal_unit=A  v_specify=off  v_priority=None  v=0 V  v_nominal_specify=off  v_nominal_value=1  v_nominal_unit=V
  Resistor4 : fl_lib/Electrical/Electrical Elements/Resistor  R=ResistanceM(2,3) Ohm  i_specify=off  i_priority=None  i=0 A  i_nominal_specify=off  i_nominal_value=1  i_nominal_unit=A  v_specify=off  v_priority=None  v=0 V  v_nominal_specify=off  v_nominal_value=1  v_nominal_unit=V
  Resistor5 : fl_lib/Electrical/Electrical Elements/Resistor  R=ResistanceM(1,3) Ohm  i_specify=off  i_priority=None  i=0 A  i_nominal_specify=off  i_nominal_value=1  i_nominal_unit=A  v_specify=off  v_priority=None  v=0 V  v_nominal_specify=off  v_nominal_value=1  v_nominal_unit=V
  Selector4 : Selector  InputPortWidth=8  IndexOptions=Index vector (dialog)  Indices=[1 6]  OutputSizes=1
  Selector5 : Selector  InputPortWidth=8  IndexOptions=Index vector (dialog)  Indices=[2 5]  OutputSizes=1
  Simulink-PS Converter : nesl_utility/Simulink-PS Converter  PhysicalDomain=network_engine_domain  SubClassName=ps_input  LeftPortType=input  RightPortType=output  PseudoPeriodic=off  Frequencies=[]  NoiseDistribution=none  NoiseParameters=[]  Unit=1  AffineConversion=off  FilteringAndDerivatives=provide  SimscapeFilterOrder=1  InputFilterTimeConstant=0.001  UdotUserProvided=0
  Simulink-PS Converter1 : nesl_utility/Simulink-PS Converter  PhysicalDomain=network_engine_domain  SubClassName=ps_input  LeftPortType=input  RightPortType=output  PseudoPeriodic=off  Frequencies=[]  NoiseDistribution=none  NoiseParameters=[]  Unit=1  AffineConversion=off  FilteringAndDerivatives=provide  SimscapeFilterOrder=1  InputFilterTimeConstant=0.001  UdotUserProvided=0
  Simulink-PS Converter2 : nesl_utility/Simulink-PS Converter  PhysicalDomain=network_engine_domain  SubClassName=ps_input  LeftPortType=input  RightPortType=output  PseudoPeriodic=off  Frequencies=[]  NoiseDistribution=none  NoiseParameters=[]  Unit=1  AffineConversion=off  FilteringAndDerivatives=provide  SimscapeFilterOrder=1  InputFilterTimeConstant=0.001  UdotUserProvided=0
  Sum1 : Sum  Inputs=|-+  InputSameDT=on  SaturateOnIntegerOverflow=on  OutDataTypeStr=Inherit: Same as first input
  Switch : Switch  Criteria=u2 > Threshold  Threshold=0.5  SaturateOnIntegerOverflow=off  InputSameDT=off
  Switch1 : Switch  Criteria=u2 > Threshold  Threshold=0.5  SaturateOnIntegerOverflow=off  InputSameDT=off
  Terminator : Terminator
  Unit Delay : UnitDelay  SampleTime=Ts  HasFrameUpgradeWarning=on
  Unit Delay1 : UnitDelay  InitialCondition=1  SampleTime=Ts  HasFrameUpgradeWarning=on
  Voltage Sensor : fl_lib/Electrical/Electrical Sensors/Voltage Sensor
  Voltage Sensor1 : fl_lib/Electrical/Electrical Sensors/Voltage Sensor
  Voltage Sensor2 : fl_lib/Electrical/Electrical Sensors/Voltage Sensor
  pole pair1 : Gain  Gain=pp
  pole pair3 : Gain  Gain=pp
  rotorzeros : Constant  Value=[0 0; 0 0;0 0]
  "   abc" : PMIOPort  Side=Left
  meas : Outport  VectorParamsAs1DForOutWhenUnconnected=off
  wires:
  Switch/1 -> [IM2_Tpark]
  ABC<->dq/1(Tstator) -> Switch/1
  Constant1/1 -> Matrice/2(park), Switch/2
  Matrice/3(speed term) -> Product2/1
  pole pair1/1 -> Matrice/1(we), Discrete-Time Integrator/1  "w_elect"
  "   w_mec"/1 -> pole pair1/1
  Matrice/2(invLdq) -> [IM2_invLdq]
  Matrice/1(Adq) -> [IM2_Adq]
  ABC<->dq/2(Trotor) -> Switch/3
  Discrete-Time Integrator/1 -> ABC<->dq/1(angle)  "theta_elect (rad)"
  [phi] -> Product1/2
  [phi] -> Gain8/1, Product4/2
  1 step prediction+2step averaging/1(Out1) -> Product2/2
  MATE/2(Ihist) -> [Ihist]
  MATE/1(Y) -> Terminator/1
  pole pair3/1 -> Bus Creator/3  "Electric torque (Nm)"
  Sum1/1 -> pole pair3/1
  Selector4/1 -> Product7/1
  Selector5/1 -> Product9/1
  Product9/1 -> Sum1/2
  Product7/1 -> Sum1/1
  Mux3/1 -> Selector4/1, Selector5/1
  Gain8/1 -> Mux3/2  "phi_dq"
  Gain9/1 -> Mux3/1  "I_dq"
  Product4/1 -> Gain9/1
  [IM2_invLdq] -> Product4/1
  Discretize/1(Ad) -> MATE/1(Ad)
  Discretize/3(Cd) -> MATE/3(Cd)
  Discretize/2(Bd) -> MATE/2(Bd)
  [IM2_Adq] -> Discretize/1(Ac)
  Matrix Concatenate1/1 -> Mat Function2/1, Discretize/2(Bc)
  Product1/1 -> Bus Creator/1  "Iabc_stator (A)"
  MATE/3(phi) -> Bus Creator/2, [phi]  "flux d-q stator d-q rotor (Wb)"
  Bus Creator/1 -> meas/1
  Unit Delay/1 -> MATE/4(u)
  [IM2_invLdq] -> Product5/2  "Linv"
  Product5/1 -> Product1/1, Discretize/3(Cc)
  rotorzeros/1 -> Mat Function1/1
  Mat Function1/1 -> Matrix Concatenate1/2
  [IM2_Tpark] -> Matrix Concatenate1/1
  [Vnode] -> Unit Delay/1
  Constant2/1 -> Discretize/4(be)
  Discretize/4(bet) -> MATE/5(bet)
  Mat Function2/1 -> Product5/1
  [omega_flux] -> MATE/7(u_speedterm)
  Discretize/5(Bdspeedterm) -> MATE/6(Bd_sp_term)
  [phi] -> 1 step prediction+2step averaging/1(In1)
  Product2/1 -> [omega_flux]
  [Va] -> Mux/1
  Gain/1 -> Demux/1
  [Ihist] -> Gain/1
  [Vc] -> Mux/3
  [Vb] -> Mux/2
  Demux/1 -> [Ia]
  Demux/2 -> [Ib]
  Demux/3 -> [Ic]
  Mux/1 -> [Vnode]
  PS-Simulink Converter/1 -> [Va]
  PS-Simulink Converter1/1 -> [Vb]
  PS-Simulink Converter2/1 -> [Vc]
  [Ia] -> Simulink-PS Converter/1
  [Ib] -> Simulink-PS Converter1/1
  [Ic] -> Simulink-PS Converter2/1
  Constant3/1 -> Switch1/2
  Switch1/1 -> [ena]
  Constant/1 -> Switch1/3
  Unit Delay1/1 -> Switch1/1
  Constant4/1 -> Unit Delay1/1
  [ena] -> Discretize/Enable
  [ena] -> ABC<->dq/Enable
  connections:
  "   abc"/RConn1 -- Phase Splitter/LConn1
  Electrical Reference/LConn1 -- Controlled Current Source/RConn2
  Controlled Current Source/LConn1 -- Voltage Sensor/LConn1 -- Phase Splitter/RConn2 -- Resistor4/LConn1 -- Resistor3/RConn1 -- Resistor/LConn1
  Electrical Reference1/LConn1 -- Resistor/RConn1
  Electrical Reference2/LConn1 -- Voltage Sensor/RConn2
  Controlled Current Source1/LConn1 -- Voltage Sensor1/LConn1 -- Phase Splitter/RConn3 -- Resistor5/RConn1 -- Resistor4/RConn1 -- Resistor1/LConn1
  Electrical Reference5/LConn1 -- Voltage Sensor1/RConn2
  Electrical Reference3/LConn1 -- Controlled Current Source1/RConn2
  Electrical Reference4/LConn1 -- Resistor1/RConn1
  Controlled Current Source2/LConn1 -- Resistor5/LConn1 -- Resistor3/LConn1 -- Resistor2/LConn1 -- Voltage Sensor2/LConn1 -- Phase Splitter/RConn1
  Electrical Reference8/LConn1 -- Voltage Sensor2/RConn2
  Electrical Reference6/LConn1 -- Controlled Current Source2/RConn2
  Electrical Reference7/LConn1 -- Resistor2/RConn1
  PS-Simulink Converter/LConn1 -- Voltage Sensor2/RConn1
  PS-Simulink Converter1/LConn1 -- Voltage Sensor/RConn1
  Voltage Sensor1/RConn1 -- PS-Simulink Converter2/LConn1
  Simulink-PS Converter/RConn1 -- Controlled Current Source2/RConn1
  Controlled Current Source/RConn1 -- Simulink-PS Converter1/RConn1
  Controlled Current Source1/RConn1 -- Simulink-PS Converter2/RConn1

== system SimScapeMATE_InductionMachine/Model Initialization ==

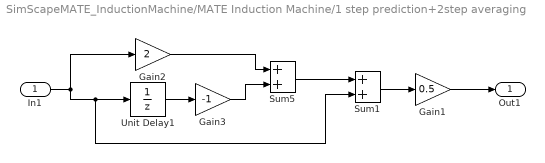
== system SimScapeMATE_InductionMachine/MATE Induction Machine/1 step prediction+2step averaging ==
  In1 : Inport
  Gain1 : Gain  Gain=0.5
  Gain2 : Gain  Gain=2
  Gain3 : Gain  Gain=-1
  Sum1 : Sum  SaturateOnIntegerOverflow=on
  Sum5 : Sum  SaturateOnIntegerOverflow=on
  Unit Delay1 : UnitDelay  SampleTime=Ts  HasFrameUpgradeWarning=on
  Out1 : Outport  VectorParamsAs1DForOutWhenUnconnected=off
  wires:
  Gain1/1 -> Out1/1
  Sum1/1 -> Gain1/1
  Sum5/1 -> Sum1/1
  Unit Delay1/1 -> Gain3/1
  Gain2/1 -> Sum5/1
  Gain3/1 -> Sum5/2
  In1/1 -> Gain2/1, Unit Delay1/1, Sum1/2

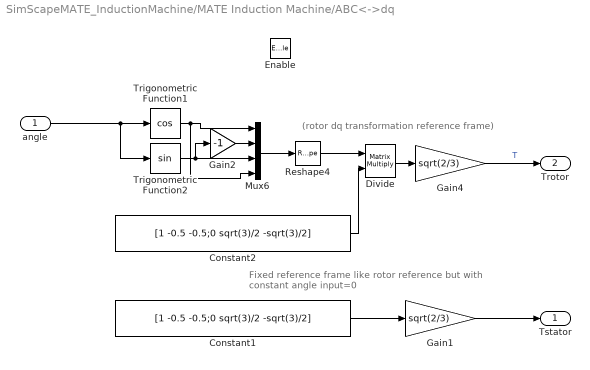
== system SimScapeMATE_InductionMachine/MATE Induction Machine/ABC<->dq ==
  note: (rotor dq transformation reference frame)
  note: Fixed reference frame
      | like rotor reference but with constant angle input=0
  angle : Inport
  Enable : EnablePort
  Constant1 : Constant  Value=[1 -0.5 -0.5;0 sqrt(3)/2 -sqrt(3)/2]
  Constant2 : Constant  Value=[1 -0.5 -0.5;0 sqrt(3)/2 -sqrt(3)/2]
  Divide : Product  Multiplication=Matrix(*)
  Gain1 : Gain  Gain=sqrt(2/3)
  Gain2 : Gain  Gain=-1
  Gain4 : Gain  Gain=sqrt(2/3)
  Mux6 : Mux
  Reshape4 : Reshape  OutputDimensionality=Customize  OutputDimensions=[2,2]
  Trigonometric Function1 : Trigonometry  Operator=cos
  Trigonometric Function2 : Trigonometry
  Tstator : Outport  VectorParamsAs1DForOutWhenUnconnected=off
  Trotor : Outport  Port=2  VectorParamsAs1DForOutWhenUnconnected=off
  wires:
  Gain2/1 -> Mux6/2
  Divide/1 -> Gain4/1
  Constant2/1 -> Divide/2
  Reshape4/1 -> Divide/1
  Mux6/1 -> Reshape4/1
  Trigonometric Function2/1 -> Mux6/3, Gain2/1
  Trigonometric Function1/1 -> Mux6/4, Mux6/1
  Constant1/1 -> Gain1/1
  angle/1 -> Trigonometric Function2/1, Trigonometric Function1/1
  Gain4/1 -> Trotor/1  "T"
  Gain1/1 -> Tstator/1

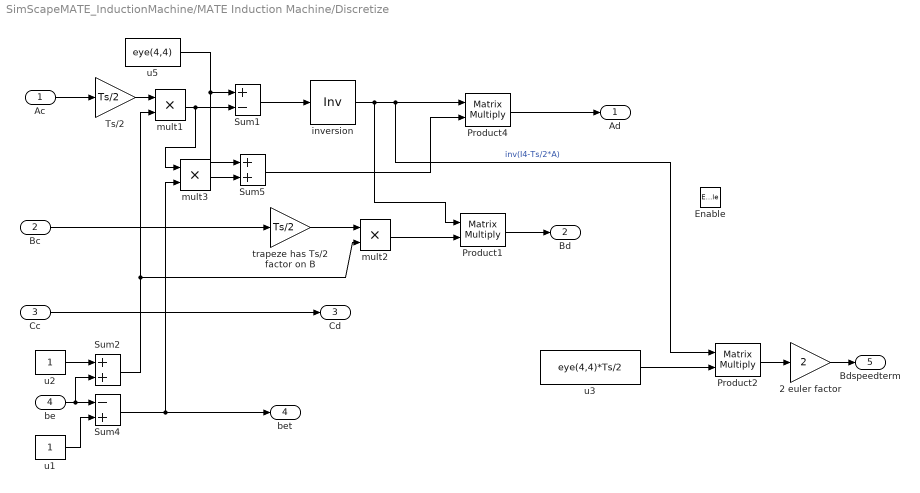
== system SimScapeMATE_InductionMachine/MATE Induction Machine/Discretize ==
  Ac : Inport
  Bc : Inport  Port=2
  Cc : Inport  Port=3
  be : Inport  Port=4
  Enable : EnablePort
  2 euler factor : Gain  Gain=2  SaturateOnIntegerOverflow=on  OutDataTypeStr=Inherit: Same as input  ParamDataTypeStr=Inherit: Same as input
  Product1 : Product  Multiplication=Matrix(*)  SaturateOnIntegerOverflow=on  OutDataTypeStr=Inherit: Same as first input
  Product2 : Product  Multiplication=Matrix(*)  SaturateOnIntegerOverflow=on  OutDataTypeStr=Inherit: Same as first input
  Product4 : Product  Multiplication=Matrix(*)  SaturateOnIntegerOverflow=on  OutDataTypeStr=Inherit: Same as first input
  Sum1 : Sum  Inputs=+-  SaturateOnIntegerOverflow=on
  Sum2 : Sum  Inputs=2  SaturateOnIntegerOverflow=on
  Sum4 : Sum  Inputs=-+  SaturateOnIntegerOverflow=on
  Sum5 : Sum  SaturateOnIntegerOverflow=on
  Ts/2 : Gain  Gain=Ts/2  SaturateOnIntegerOverflow=on  OutDataTypeStr=Inherit: Same as input  ParamDataTypeStr=Inherit: Same as input
  inversion : Product  Inputs=/  Multiplication=Matrix(*)  RndMeth=Zero
  mult1 : Product
  mult2 : Product
  mult3 : Product
  trapeze has Ts/2 factor on B : Gain  Gain=Ts/2  SaturateOnIntegerOverflow=on  OutDataTypeStr=Inherit: Same as input  ParamDataTypeStr=Inherit: Same as input
  u1 : Constant
  u2 : Constant
  u3 : Constant  Value=eye(4,4)*Ts/2
  u5 : Constant  Value=eye(4,4)
  Ad : Outport  VectorParamsAs1DForOutWhenUnconnected=off
  Bd : Outport  Port=2  VectorParamsAs1DForOutWhenUnconnected=off
  Cd : Outport  Port=3  VectorParamsAs1DForOutWhenUnconnected=off
  bet : Outport  Port=4  VectorParamsAs1DForOutWhenUnconnected=off
  Bdspeedterm : Outport  Port=5  VectorParamsAs1DForOutWhenUnconnected=off
  wires:
  Sum1/1 -> inversion/1
  Ac/1 -> Ts/2/1
  Product1/1 -> Bd/1
  Sum5/1 -> Product4/2
  u5/1 -> Sum1/1, Sum5/1
  Product4/1 -> Ad/1
  Ts/2/1 -> mult1/1
  trapeze has Ts/2 factor on B/1 -> mult2/1
  inversion/1 -> Product1/1, Product2/1, Product4/1  "inv(I4-Ts/2*A)"
  Cc/1 -> Cd/1
  Bc/1 -> trapeze has Ts/2 factor on B/1
  u2/1 -> Sum2/1
  be/1 -> Sum2/2, Sum4/1
  u1/1 -> Sum4/2
  mult1/1 -> Sum1/2, mult3/1
  mult3/1 -> Sum5/2
  Sum4/1 -> mult3/2, bet/1
  mult2/1 -> Product1/2
  u3/1 -> Product2/2
  Sum2/1 -> mult1/2, mult2/2
  Product2/1 -> 2 euler factor/1
  2 euler factor/1 -> Bdspeedterm/1

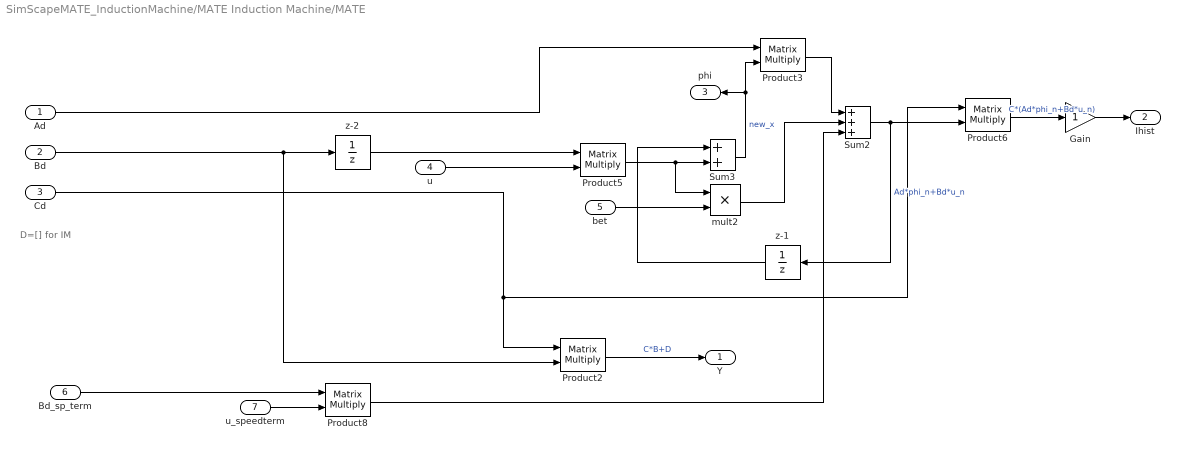
== system SimScapeMATE_InductionMachine/MATE Induction Machine/MATE ==
  note: D=[] for IM
  Ad : Inport
  Bd : Inport  Port=2
  Cd : Inport  Port=3
  u : Inport  Port=4
  bet : Inport  Port=5
  Bd_sp_term : Inport  Port=6
  u_speedterm : Inport  Port=7
  Gain : Gain
  Product{2..3,5..6,8} (5 alike) : Product  Multiplication=Matrix(*)  SaturateOnIntegerOverflow=on  OutDataTypeStr=Inherit: Same as first input
  Sum2 : Sum  Inputs=+++  SaturateOnIntegerOverflow=on
  Sum3 : Sum  SaturateOnIntegerOverflow=on
  mult2 : Product
  z-1 : UnitDelay  SampleTime=Ts  HasFrameUpgradeWarning=on
  z-2 : UnitDelay  SampleTime=Ts  HasFrameUpgradeWarning=on
  Y : Outport  VectorParamsAs1DForOutWhenUnconnected=off
  Ihist : Outport  Port=2  VectorParamsAs1DForOutWhenUnconnected=off
  phi : Outport  Port=3  VectorParamsAs1DForOutWhenUnconnected=off
  wires:
  Cd/1 -> Product2/1, Product6/1
  Product2/1 -> Y/1  "C*B+D"
  Product5/1 -> Sum3/2, mult2/1
  Product3/1 -> Sum2/1
  Sum2/1 -> z-1/1, Product6/2  "Ad*phi_n+Bd*u_n"
  Product6/1 -> Gain/1  "C*(Ad*phi_n+Bd*u_n)"
  Ad/1 -> Product3/1
  Bd/1 -> Product2/2, z-2/1
  u/1 -> Product5/2
  Gain/1 -> Ihist/1
  z-1/1 -> Sum3/1
  bet/1 -> mult2/2
  Bd_sp_term/1 -> Product8/1
  u_speedterm/1 -> Product8/2
  Product8/1 -> Sum2/3
  mult2/1 -> Sum2/2
  Sum3/1 -> phi/1, Product3/2  "new_x"
  z-2/1 -> Product5/1

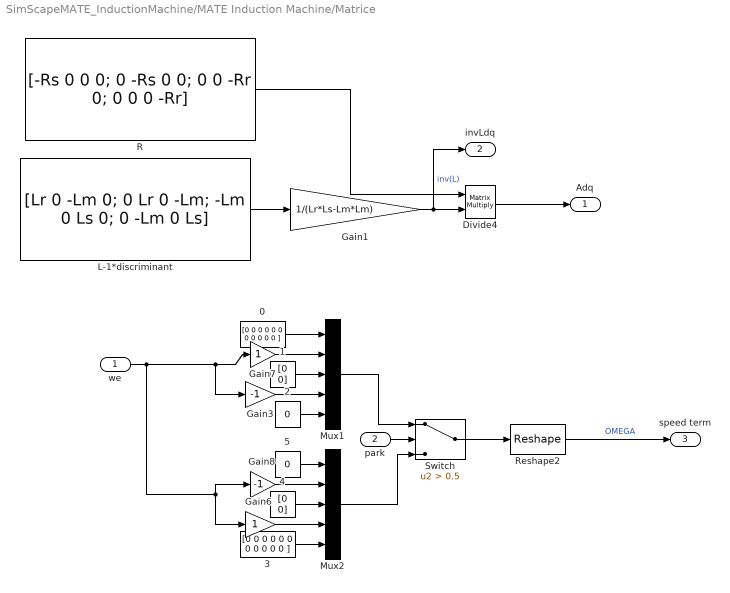
== system SimScapeMATE_InductionMachine/MATE Induction Machine/Matrice ==
  we : Inport
  park : Inport  Port=2
  0 : Constant  Value=[0 0 0 0 0 0 0 0 0 0 0 ]
  1 : Constant  Value=[0 0]
  2 : Constant  Value=0
  3 : Constant  Value=[0 0 0 0 0 0 0 0 0 0 0 ]
  4 : Constant  Value=[0 0]
  5 : Constant  Value=0
  Divide4 : Product  Multiplication=Matrix(*)
  Gain1 : Gain  Gain=1/(Lr*Ls-Lm*Lm)
  Gain3 : Gain  Gain=-1
  Gain6 : Gain
  Gain7 : Gain
  Gain8 : Gain  Gain=-1
  L-1*discriminant : Constant  Value="[Lr 0 -Lm 0; 0 Lr 0 -Lm; -Lm 0  Ls  0;  0  -Lm  0  Ls]"
  Mux1 : Mux  Inputs=[11 1 2 1 1]
  Mux2 : Mux  Inputs=[1 1 2 1 11]
  R : Constant  Value="[-Rs 0 0 0; 0 -Rs 0 0; 0 0  -Rr  0;  0  0  0  -Rr]"
  Reshape2 : Reshape  OutputDimensionality=Customize  OutputDimensions=[4,4]
  Switch : Switch  Criteria=u2 > Threshold  Threshold=0.5  SaturateOnIntegerOverflow=off  InputSameDT=off
  Adq : Outport  VectorParamsAs1DForOutWhenUnconnected=off
  invLdq : Outport  Port=2  VectorParamsAs1DForOutWhenUnconnected=off
  speed term : Outport  Port=3  VectorParamsAs1DForOutWhenUnconnected=off
  wires:
  3/1 -> Mux2/5
  5/1 -> Mux2/1
  Mux2/1 -> Switch/3
  Mux1/1 -> Switch/1
  Switch/1 -> Reshape2/1
  park/1 -> Switch/2
  we/1 -> Gain3/1, Gain7/1, Gain8/1, Gain6/1
  Gain6/1 -> Mux2/4
  4/1 -> Mux2/3
  Gain8/1 -> Mux2/2
  Gain1/1 -> invLdq/1, Divide4/2  "inv(L)"
  0/1 -> Mux1/1
  Gain3/1 -> Mux1/4
  Divide4/1 -> Adq/1
  1/1 -> Mux1/3
  2/1 -> Mux1/5
  Gain7/1 -> Mux1/2
  R/1 -> Divide4/1
  Reshape2/1 -> speed term/1  "OMEGA"
  L-1*discriminant/1 -> Gain1/1
